simulink model "template"  (R2019b)
settings: Solver=VariableStepAuto  StartTime=0.0  StopTime=40  RelTol=1e-3
values from neighbouring files (symbols this model uses):
  a1 = rho * D^4 * alpha1    (= 0.000388302366464)    [data.m]
  a2 = -rho * D^3 * alpha2 * (1 - omega)    (= 0.0037030698432)    [data.m]
  alpha1 = 0.0113    [data.m]
  alpha2 = -0.0091    [data.m]
  D = 0.076    [data.m]
  dead_zone_limit = 31.5    [data.m]
  n_max = 340    [data.m]
  omega = 0.1    [data.m]
settings Model: Creator=ric  LastModifiedBy=ric

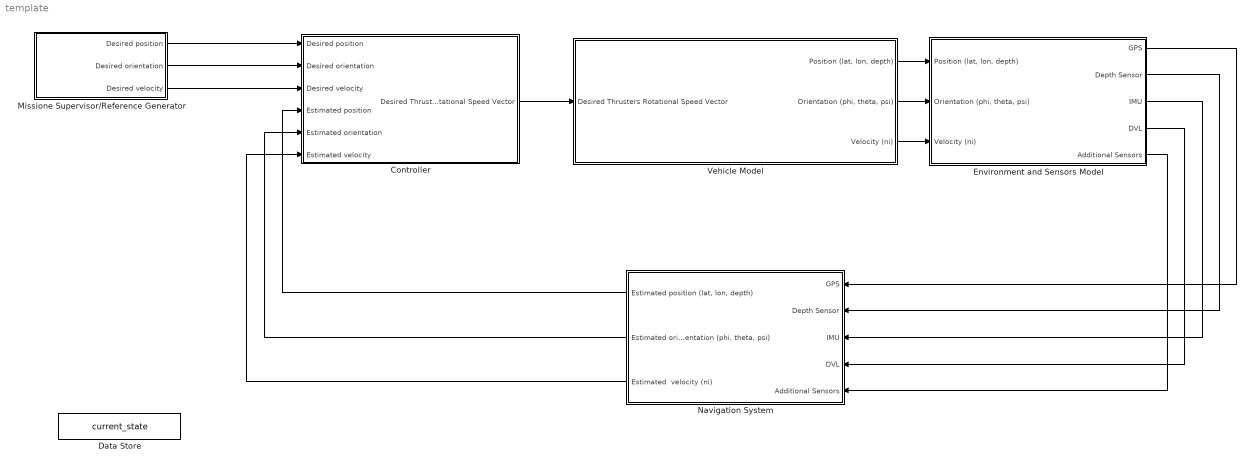
== system template ==
  Controller : Subsystem
  Data Store : DataStoreMemory  DataStoreName=current_state  ReadBeforeWriteMsg=warning  WriteAfterWriteMsg=warning  WriteAfterReadMsg=warning  ShowAdditionalParam=off
  Environment and Sensors Model : Subsystem
  Missione Supervisor/Reference Generator : Subsystem
  Navigation System : Subsystem
  Vehicle Model : Subsystem
  wires:
  Vehicle Model/1("Position (lat, lon, depth)") -> Environment and Sensors Model/1("Position (lat, lon, depth)")
  Vehicle Model/2("Orientation (phi, theta, psi)") -> Environment and Sensors Model/2("Orientation (phi, theta, psi)")
  Vehicle Model/3(Velocity (ni)) -> Environment and Sensors Model/3(Velocity (ni))
  Environment and Sensors Model/1(GPS) -> Navigation System/1(GPS)
  Environment and Sensors Model/2(Depth Sensor) -> Navigation System/2(Depth Sensor)
  Environment and Sensors Model/3(IMU) -> Navigation System/3(IMU)
  Environment and Sensors Model/4(DVL) -> Navigation System/4(DVL)
  Environment and Sensors Model/5(Additional Sensors) -> Navigation System/5(Additional Sensors)
  Controller/1(Desired Thrusters Rotational Speed Vector) -> Vehicle Model/1(Desired Thrusters Rotational Speed Vector)
  Navigation System/1("Estimated position (lat, lon, depth)") -> Controller/4(Estimated position)
  Navigation System/2("Estimated orientation (phi, theta, psi)") -> Controller/5(Estimated orientation)
  Navigation System/3(Estimated  velocity (ni)) -> Controller/6(Estimated velocity)
  Missione Supervisor/Reference Generator/1(Desired position) -> Controller/1(Desired position)
  Missione Supervisor/Reference Generator/2(Desired orientation) -> Controller/2(Desired orientation)
  Missione Supervisor/Reference Generator/3(Desired velocity) -> Controller/3(Desired velocity)

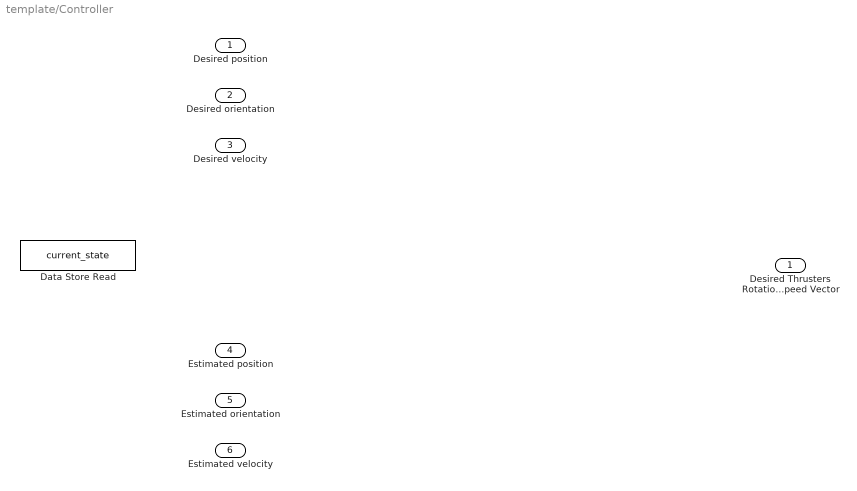
== system template/Controller ==
  Desired position : Inport
  Desired orientation : Inport  Port=2
  Desired velocity : Inport  Port=3
  Estimated position : Inport  Port=4
  Estimated orientation : Inport  Port=5
  Estimated velocity : Inport  Port=6
  Data Store Read : DataStoreRead  DataStoreName=current_state  SampleTime=0.001
  Desired Thrusters Rotational Speed Vector : Outport

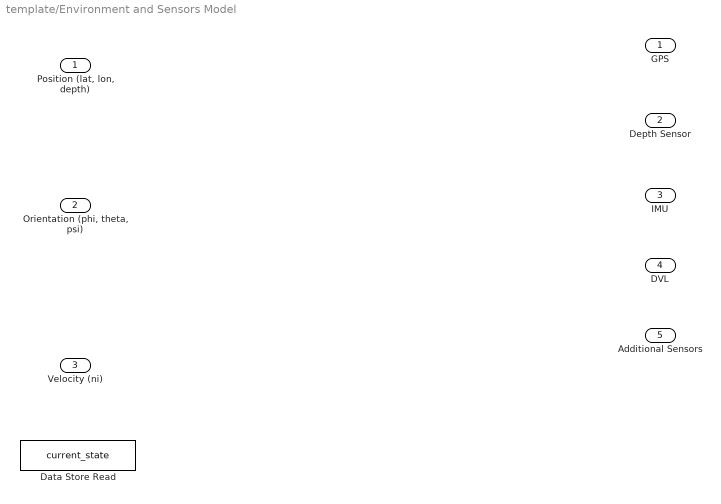
== system template/Environment and Sensors Model ==
  "Position (lat, lon, depth)" : Inport
  "Orientation (phi, theta, psi)" : Inport  Port=2
  Velocity (ni) : Inport  Port=3
  Data Store Read : DataStoreRead  DataStoreName=current_state  SampleTime=0.001
  GPS : Outport
  Depth Sensor : Outport  Port=2
  IMU : Outport  Port=3
  DVL : Outport  Port=4
  Additional Sensors : Outport  Port=5

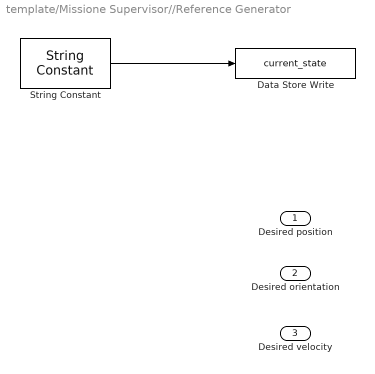
== system template/Missione Supervisor//Reference Generator ==
  Data Store Write : DataStoreWrite  DataStoreName=current_state
  String Constant : StringConstant  String="\"Init\""
  Desired position : Outport
  Desired orientation : Outport  Port=2
  Desired velocity : Outport  Port=3
  wires:
  String Constant/1 -> Data Store Write/1

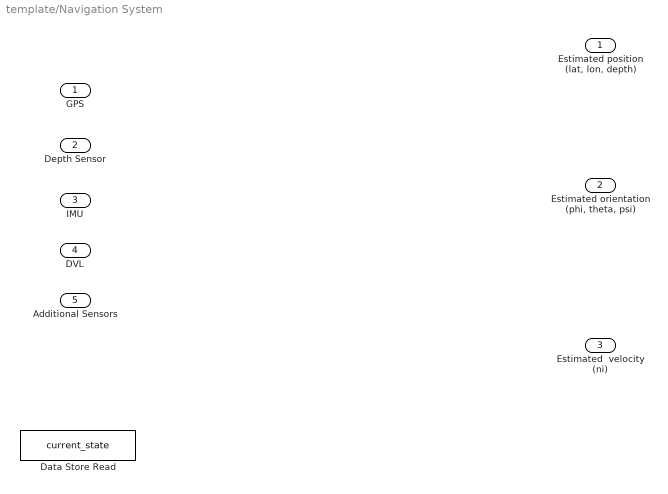
== system template/Navigation System ==
  GPS : Inport
  Depth Sensor : Inport  Port=2
  IMU : Inport  Port=3
  DVL : Inport  Port=4
  Additional Sensors : Inport  Port=5
  Data Store Read : DataStoreRead  DataStoreName=current_state  SampleTime=0.001
  "Estimated position (lat, lon, depth)" : Outport
  "Estimated orientation (phi, theta, psi)" : Outport  Port=2
  Estimated  velocity (ni) : Outport  Port=3

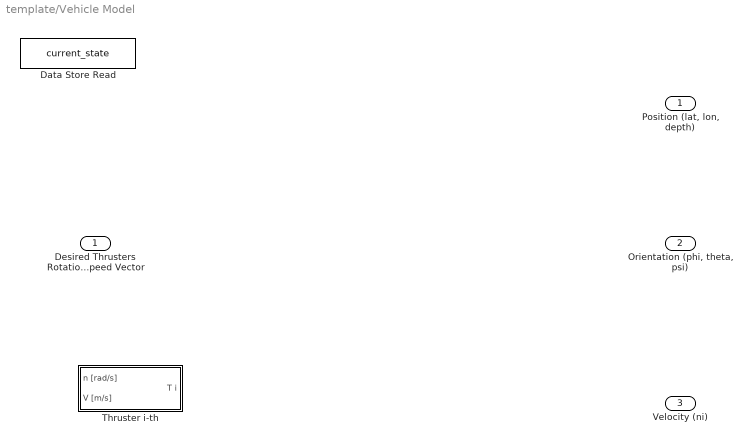
== system template/Vehicle Model ==
  Desired Thrusters Rotational Speed Vector : Inport
  Data Store Read : DataStoreRead  DataStoreName=current_state  SampleTime=0.001
  Thruster i-th : Subsystem
  "Position (lat, lon, depth)" : Outport
  "Orientation (phi, theta, psi)" : Outport  Port=2
  Velocity (ni) : Outport  Port=3

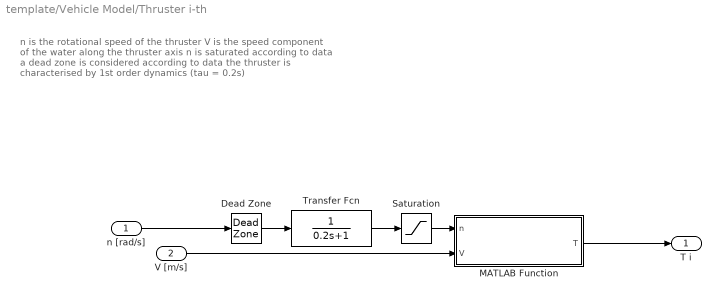
== system template/Vehicle Model/Thruster i-th ==
  note: n is the rotational speed of the thruster
      | V is the speed component of the water along the thruster axis
      |
      | n is saturated according to data
      | a dead zone is considered according to data
      | the thruster is characterised by 1st order dynamics (tau = 0.2s)
  n [rad/s] : Inport
  V [m/s] : Inport  Port=2
  Dead Zone : DeadZone  LowerValue=-dead_zone_limit  UpperValue=dead_zone_limit  SaturateOnIntegerOverflow=on
  MATLAB Function : MATLAB Function  TreatAsAtomicUnit=on
  Saturation : Saturate  UpperLimit=n_max  LowerLimit=-n_max
  Transfer Fcn : TransferFcn  Denominator=[0.2 1]
  T i : Outport
  wires:
  V [m/s]/1 -> MATLAB Function/2(V)
  Saturation/1 -> MATLAB Function/1(n)
  Transfer Fcn/1 -> Saturation/1
  Dead Zone/1 -> Transfer Fcn/1
  n [rad/s]/1 -> Dead Zone/1
  MATLAB Function/1(T) -> T i/1

== matlab function template/Vehicle Model/Thruster i-th/MATLAB Function ==
  data: n input; T output; V input; D parameter; omega parameter; a1 parameter; a2 parameter; alpha1 parameter; alpha2 parameter
function T = thrusterModel(n, V, D, omega, a1, a2, alpha1, alpha2)

Va = (1-omega) * V;     % Advancement velocity at the propeller
J0 = Va/(n*D);          % Advancement Coefficient

if J0 > -alpha1/alpha2  % Out of linearity domain (right side)
    T = 0;              % A null generated thrust is assumed
    
elseif J0 < 0           % Out of linearity domain (left side)
    T = a1*abs(n)*n;    % Bollard thrust is assumed

else                    % Within the linearity domain
    T = a1*abs(n)*n - a2*abs(n)*V;
end
